simulink model "myevapmods"  (R2021a)
settings: Solver=VariableStepAuto  StartTime=0.0  StopTime=100  RelTol=1e-3
settings Model: Creator=Arman  LastModifiedBy=49152
settings SolverCC: AlgebraicLoopSolver=TrustRegion
settings DebuggingCC: SFMachineParentedDataDiag=warning

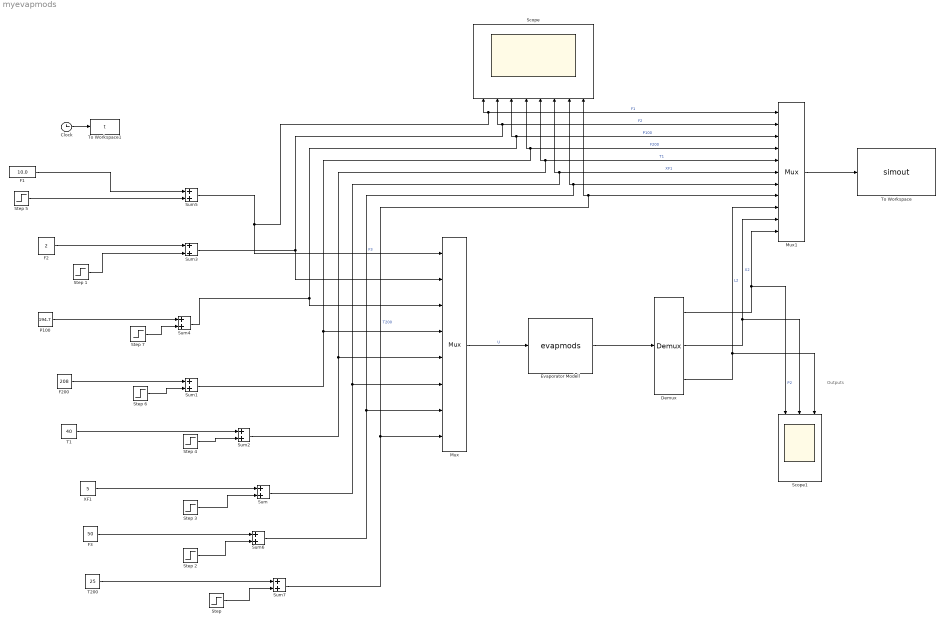
== system myevapmods ==
  note: Outputs
  Clock : Clock
  Demux : Demux  Outputs=[1,1,1]
      settings: DisplayOption=none
  "Evaporator Modell " : S-Function  FunctionName=evapmods  SFunctionDeploymentMode=off  EnableBusSupport=off
  F1 : Constant  Value=10.0
  F2 : Constant  Value=2
  F200 : Constant  Value=208
  F3 : Constant  Value=50
  Mux : Mux  Inputs=8
      settings: DisplayOption=signals
  Mux1 : Mux  Inputs=11
      settings: DisplayOption=signals
  P100 : Constant  Value=194.7
  Scope : Scope  NumInputPorts=8
  Scope1 : Scope  NumInputPorts=3
  "Step " : Step  Time=10  After=0.80  SampleTime=1
  Step 1 : Step  Time=0  After=0  SampleTime=0
  Step 2 : Step  Time=0  After=0.0  SampleTime=0
  Step 3 : Step  Time=0  After=0  SampleTime=0
  Step 4 : Step  Time=0  After=0.0  SampleTime=0
  Step 5 : Step  Time=0  After=0  SampleTime=0
  Step 6 : Step  Time=0  After=0.0  SampleTime=0
  Step 7 : Step  Time=0  After=0.00  SampleTime=0
  Sum{,1..7} (8 alike) : Sum  InputSameDT=on  SaturateOnIntegerOverflow=on  OutDataTypeStr=Inherit: Same as first input
  T1 : Constant  Value=40
  T200 : Constant  Value=25
  To Workspace : ToWorkspace  VariableName=simout  SampleTime=0.5
  To Workspace1 : ToWorkspace  VariableName=t  SampleTime=0.5
  XF1 : Constant  Value=5
  wires:
  Clock/1 -> To Workspace1/1
  Mux1/1 -> To Workspace/1
  Mux/1 -> "Evaporator Modell "/1  "U"
  Demux/1 -> Scope1/1, Mux1/11  "P2"
  "Evaporator Modell "/1 -> Demux/1
  Demux/2 -> Scope1/2, Mux1/10  "X2"
  Demux/3 -> Mux1/9, Scope1/3  "L2"
  F200/1 -> Sum1/1
  T1/1 -> Sum2/1
  XF1/1 -> Sum/1
  T200/1 -> Sum7/1
  P100/1 -> Sum4/1
  F3/1 -> Sum6/1
  Sum5/1 -> Mux/1, Mux1/1, Scope/1  "F1"
  Sum3/1 -> Mux/2, Mux1/2, Scope/2  "F2"
  Sum4/1 -> Mux1/3, Scope/3, Mux/3  "P100"
  Sum1/1 -> Mux1/4, Scope/4, Mux/4  "F200"
  Sum2/1 -> Mux/5, Mux1/5, Scope/5  "T1"
  Sum/1 -> Mux1/6, Scope/6, Mux/6  "XF1"
  Sum6/1 -> Mux1/7, Scope/7, Mux/7  "F3"
  Sum7/1 -> Scope/8, Mux1/8, Mux/8  "T200"
  F1/1 -> Sum5/1
  F2/1 -> Sum3/1
  Step 4/1 -> Sum2/2
  Step 3/1 -> Sum/2
  Step 2/1 -> Sum6/2
  "Step "/1 -> Sum7/2
  Step 6/1 -> Sum1/2
  Step 7/1 -> Sum4/2
  Step 1/1 -> Sum3/2
  Step 5/1 -> Sum5/2
